simulink model "Rocket_Model"  (R2023a)
settings: Solver=ode23t  StartTime=0.0  StopTime=100  RelTol=1e-2
settings Model: Creator=jxs210080  LastModifiedBy=jxs210080

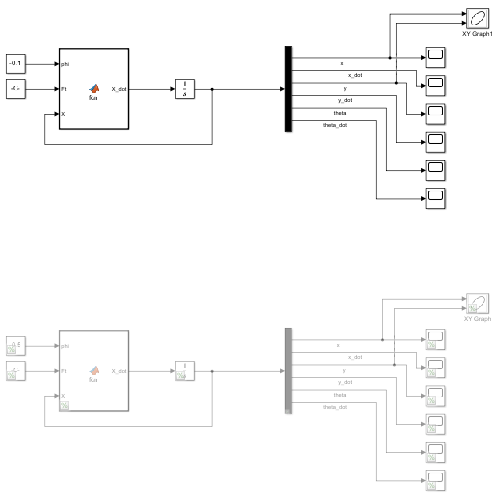
[thumbnail: Simulink's stored preview of the top-level diagram]
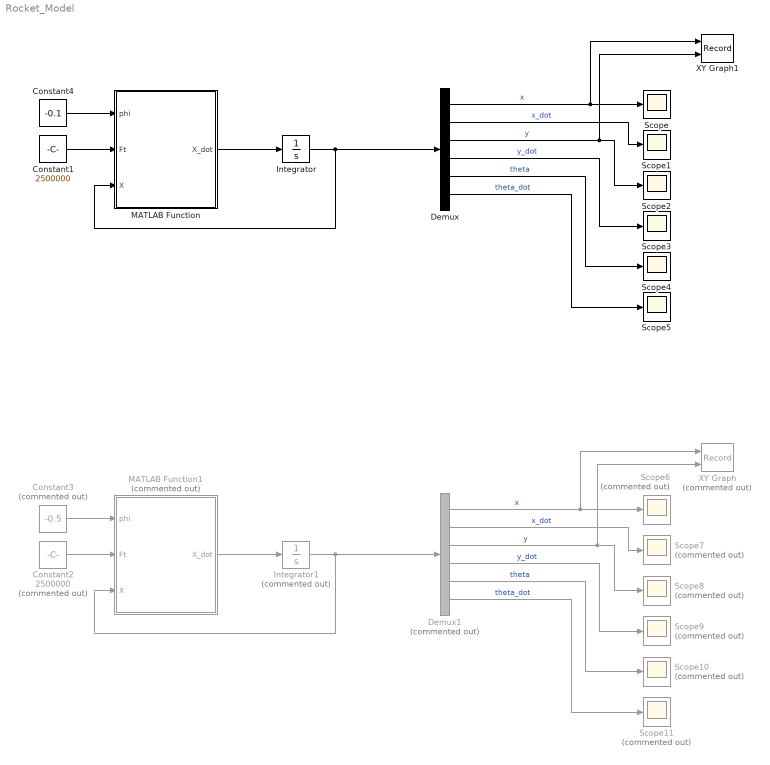
== system Rocket_Model ==
  Constant1 : Constant  Value=2500000
  Constant2 : Constant  Commented=on  Value=2500000
  Constant3 : Constant  Commented=on  Value=-0.5
  Constant4 : Constant  Value=-0.1
  Demux : Demux  Outputs=6
  Demux1 : Demux  Commented=on  Outputs=6
  Integrator : Integrator  InitialCondition=[0; 0; 0; 0; 0; 0]
  Integrator1 : Integrator  Commented=on  InitialCondition=[0; 0; 0; 0; 0; 0]
  MATLAB Function : MATLAB Function  TreatAsAtomicUnit=on
  MATLAB Function1 : MATLAB Function  Commented=on  TreatAsAtomicUnit=on
  Scope{,1..5} (6 alike) : Scope
  Scope{6..11} (6 alike) : Scope  Commented=on
  XY Graph : Record  Commented=on  FileSettingsInternal="{\"entries\":[{\"content\":{\"excelSettings\":{\"content\":{},\"type\":\"Streamout.ExcelSettings\"}},\"type\":\"Streamout.FileSettingStorage\",\"uuid\":\"\"}],\"packageUris\":[\"http:\\/\\/schema.mathworks.com\\/mf0\\/streamout_blocks\\/R2020a\"],\"version\":\"1.0\"}"  Layout=[1 1]  SignalsInternal="{\"entries\":[{\"content\":{},\"type\":\"RecordBlkView.InputSignals\",\"uuid\":\"\"}],\"packageUris\":[\"http:\\/\\/schema.mathworks.com\\/mf0\\/streamout_blocks\\/R2020a\"],\"version\":\"1.0\"}"  VisualizationBindings="{\"xyplotplugin\":{\"info\":[{\"series\":[],\"subplotID\":1}]}}"  CompatibilityTag=XY
  XY Graph1 : Record  FileSettingsInternal="{\"entries\":[{\"content\":{\"excelSettings\":{\"content\":{},\"type\":\"Streamout.ExcelSettings\"}},\"type\":\"Streamout.FileSettingStorage\",\"uuid\":\"\"}],\"packageUris\":[\"http:\\/\\/schema.mathworks.com\\/mf0\\/streamout_blocks\\/R2020a\"],\"version\":\"1.0\"}"  Layout=[1 1]  SignalsInternal="{\"entries\":[{\"content\":{\"signals\":[{\"content\":{\"blockPath\":[],\"dimensions\":[1,1],\"domain\":\"\",\"lineColor\":\"#22b573\",\"port\":1,\"sid\":[\"\"],\"signalID\":2678,\"signalName\":\"x\"},\"type\":\"RecordBlkView.Signal\",\"uuid\":\"\"},{\"content\":{\"blockPath\":[],\"dimensions\":[1,1],\"domain\":\"\",\"lineColor\":\"#0072bd\",\"port\":2,\"sid\":[\"\"],\"signalID\":2682,\"signalName\":\"y\"},\"type\":\"RecordBlkView.Signal\",\"uuid\":\"\"}]},\"type\":\"RecordBlkView.InputSignals\",\"uuid\":\"\"}],\"packageUris\":[\"http:\\/\\/schema.mathworks.com\\/mf0\\/streamout_blocks\\/R2020a\"],\"version\":\"1.0\"}"  VisualizationBindings="{\"xyplotplugin\":{\"info\":[{\"series\":[],\"subplotID\":1}]}}"  CompatibilityTag=XY
  wires:
  MATLAB Function/1(X_dot) -> Integrator/1
  Integrator/1 -> MATLAB Function/3(X), Demux/1
  Demux/1 -> XY Graph1/1, Scope/1  "x"
  Demux/2 -> Scope1/1  "x_dot"
  Demux/3 -> XY Graph1/2, Scope2/1  "y"
  Demux/4 -> Scope3/1  "y_dot"
  Demux/5 -> Scope4/1  "theta"
  Demux/6 -> Scope5/1  "theta_dot"
  Demux1/2 -> Scope7/1  "x_dot"
  Demux1/6 -> Scope11/1  "theta_dot"
  Demux1/1 -> XY Graph/1, Scope6/1  "x"
  MATLAB Function1/1(X_dot) -> Integrator1/1
  Integrator1/1 -> MATLAB Function1/3(X), Demux1/1
  Demux1/3 -> XY Graph/2, Scope8/1  "y"
  Demux1/4 -> Scope9/1  "y_dot"
  Demux1/5 -> Scope10/1  "theta"
  Constant2/1 -> MATLAB Function1/2(Ft)
  Constant3/1 -> MATLAB Function1/1(phi)
  Constant4/1 -> MATLAB Function/1(phi)
  Constant1/1 -> MATLAB Function/2(Ft)

== matlab function Rocket_Model/MATLAB Function ==
  data: phi input; X_dot output; Ft input; X input
function X_dot  = fcn(phi, Ft, X)

g = 9.81;
l = 100;
M = 1000;

X_dot = [X(2); (Ft*sin(phi)*cos(X(5)) - sin(X(5))*Ft*cos(phi))/M; X(4); (Ft*cos(phi)*cos(X(5)) + Ft*sin(phi)*sin(X(5)))/M - g; X(6); 6*(Ft*sin(phi)/(M*l))];


end

== matlab function Rocket_Model/MATLAB Function1 ==
  data: phi input; X_dot output; Ft input; X input
function X_dot  = fcn(phi, Ft, X)

g = 9.81;
l = 100;
M = 1000;

Ft0 = Ft;
theta0 = X(5);
phi0 = phi;

A = [0 1 0 0 0 0; 0 0 0 0 Ft0*cos(theta0-phi0)/M 0; 0 0 0 1 0 0; 0 0 0 0 -Ft0*sin(theta0+phi0)/M 0; 0 0 0 0 0 1; 0 0 0 0 0 0];
B = [0 0; sin(theta0+phi0)/M Ft0*cos(theta0+phi0)/M; 0 0; cos(theta0+phi0)/M -Ft0*sin(theta0+phi0)/M; 0 0; (-6/M*l)*sin(phi0) -6*(Ft0/M*l)*cos(phi0)];

X_dot = A*X + B*[Ft; phi];

end
